simulink model "SAR_Heavy_Mapper_SITL_3D_v1"  (R2025b)
settings: Solver=ode4  StartTime=0.0  StopTime=inf  FixedStep=1/60  RelTol=1e-3
libraries: dspnetwork x4, sim3dlib x1, uavsim3dlib x1
settings Model: Creator=User  LastModifiedBy=User

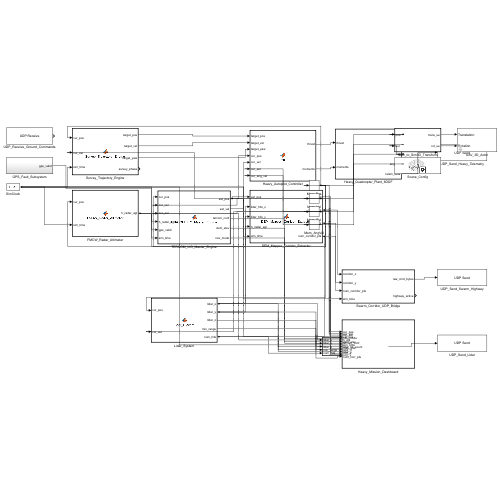
[thumbnail: Simulink's stored preview of the top-level diagram]
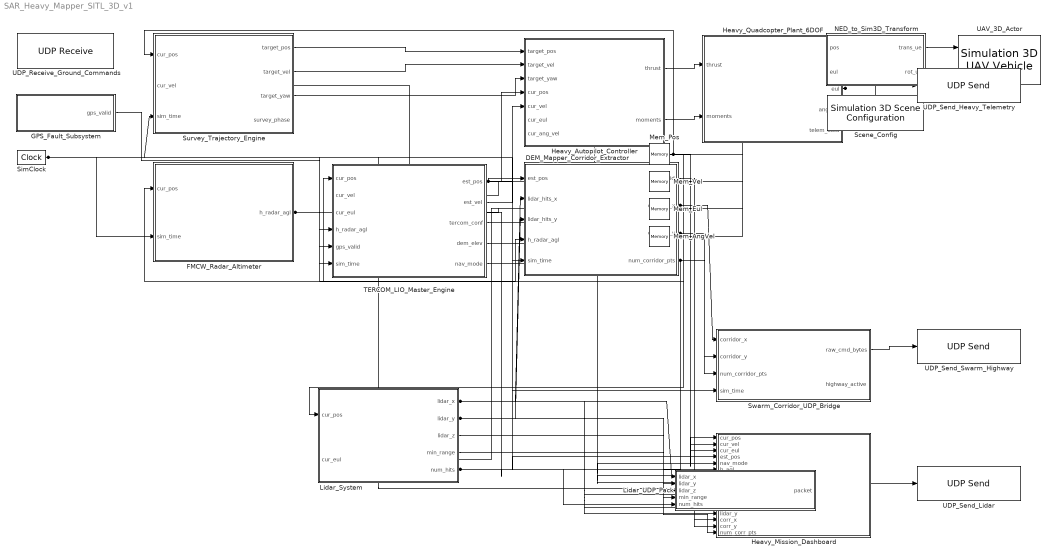
== system SAR_Heavy_Mapper_SITL_3D_v1 ==
  DEM_Mapper_Corridor_Extractor : MATLAB Function  TreatAsAtomicUnit=on
  FMCW_Radar_Altimeter : MATLAB Function  TreatAsAtomicUnit=on
  GPS_Fault_Subsystem : Subsystem
  Heavy_Autopilot_Controller : MATLAB Function  TreatAsAtomicUnit=on
  Heavy_Mission_Dashboard : MATLAB Function  TreatAsAtomicUnit=on
  Heavy_Quadcopter_Plant_6DOF : MATLAB Function  TreatAsAtomicUnit=on
  Lidar_System : MATLAB Function  TreatAsAtomicUnit=on
  Lidar_UDP_Pack : MATLAB Function  TreatAsAtomicUnit=on
  Mem_AngVel : Memory  InitialCondition=[0; 0; 0]
  Mem_Eul : Memory  InitialCondition=[0; 0; 0]
  Mem_Pos : Memory  InitialCondition=[0; 0; -70]
  Mem_Vel : Memory  InitialCondition=[0; 0; 0]
  NED_to_Sim3D_Transform : MATLAB Function  TreatAsAtomicUnit=on
  Scene_Config : sim3dlib/Simulation 3D Scene Configuration  Priority=0  ProjectFormat=Default Scenes  SceneDesc=US city block  ProjectName=D:\MLAB\toolbox\shared\sim3d_projects\automotive_project_windows\UE\WindowsNoEditor\VehicleSimulation.exe  ScenePath=/Game/Maps/USCityBlock  EnableOpenDRIVE=off  vehTagList={'Custom';'Scene Origin'}  vehTag=Scene Origin  AttachedCameraRelativeTranslation=[0 0 0]  FreeCameraDefaultInitialTranslation=[-6, 0, 2]  AttachedCameraRelativeRotation=[0 0 0]  FreeCameraDefaultInitialRotation=[0, -15, 0]  ViewpointName=Custom  FreeCameraInitialTranslation=[0, 0, 0]  ViewpointTranslation=[0, 0, 0]  FreeCameraInitialRotation=[0, 0, 0]  ViewpointRotation=[0, 0, 0]  OpVisEn=off  Ts=1/60  EnableWindow=on  EnableRemoteAccess=off  EnableWeather=off  SunAzimuth=90  SunAltitude=40.0  EnableGeospatialSun=off  Latitude=0  Longitude=0  Date=2023-01-01  Time=10:30:00  GeoTimeZone=-5.0  SunDaylightSaving=off  wind=1  clouds=10  EnableVolumetricClouds=off  CloudCoverage=0  CloudAltitude=6  fog=0  rain=0  RaindropsEffect=off  SnowDensity=0  EnableGeospatial=off  TilesetSource=Earth terrain  UseTrueOrigin=off  OriginHeight=200  OriginLatitude=40.744652  OriginLongitude=-73.988864  MapStyle=Aerial  AdditionalAssetIDs=[]  UseAdvancedSunSky=off  SolarTime=11  TimeZone=-5  Day=21  Month=9  Year=2022  UseDaylightSavingTime=on  DSTStartDay=10  DSTStartMonth=3  DSTEndDay=3  DSTEndMonth=11  DSTSwitchHour=2  sensorTag=MainCamera1  sensorId=1  sensorName=MainCamera1  mountLoc=Origin  offsetFlag=off  tmountOffset=[0, 0, 0]  rmountOffset=[0, 0, 0]  HorizontalResolution=1280  VerticalResolution=720  HorizontalFOV=60  mountPoint=[0 0 0]  mountOrientation=[0 0 0]  aMode=4  ID=1  GeoTrigger=Inactive  ViewNameList={'Custom'}  ViewTranslationList={'[0 0 0]'}  ViewRotationList={'[0 0 0]'}
      settings: LibrarySourceBlock=uavsim3dlib/Simulation 3D Scene Configuration
  SimClock : DigitalClock  SampleTime=1/60
  Survey_Trajectory_Engine : MATLAB Function  TreatAsAtomicUnit=on
  Swarm_Corridor_UDP_Bridge : MATLAB Function  TreatAsAtomicUnit=on
  TERCOM_LIO_Master_Engine : MATLAB Function  TreatAsAtomicUnit=on
  UAV_3D_Actor : uavsim3dlib/Simulation 3D UAV Vehicle  Priority=-1  Mesh=Quadrotor  MeshPath=/MathWorksUAVContent/UAVs/HexaRotorUAV/HexaRotor.HexaRotor  Color=Black  ActorName=SimulinkVehicle1  UseGlobalFrame=off  InitialTranslation=[0 0 0]  InitialRotation=[0 0 0]  InitialTranslationGlobal=[0 0 0]  InitialGeoOrigin=[0 0 0]  InitialRotationGlobal=[0 0 0]  SampleTime=-1  ActorType=SimulinkVehicle  ID=1  aMode=4  ActorTag=SimulinkVehicle1
  UDP_Receive_Ground_Commands : dspnetwork/UDP Receive  localURL='0.0.0.0'  localPort=6001  remoteURL='0.0.0.0'  remotePort=-1  recvBufferSize=8192  dims=255  signalDatatype=uint8  isComplex=off  isVarSize=on  showBlockingTime=off  blockingTime=0  sampletime=1  blockPlatform=[]
  UDP_Send_Heavy_Telemetry : dspnetwork/UDP Send  remoteURL='127.0.0.1'  remotePort=6002  localURL='0.0.0.0'  localPortSource=Automatically determine  localPort=2048  sendBufferSize=8192  sampletime=-1  blockPlatform=[]  separateLengthPort=0
  UDP_Send_Lidar : dspnetwork/UDP Send  remoteURL='127.0.0.1'  remotePort=5003  localURL='0.0.0.0'  localPortSource=Automatically determine  localPort=2048  sendBufferSize=8192  sampletime=-1  blockPlatform=[]  separateLengthPort=0
  UDP_Send_Swarm_Highway : dspnetwork/UDP Send  remoteURL='127.0.0.1'  remotePort=5001  localURL='0.0.0.0'  localPortSource=Automatically determine  localPort=2048  sendBufferSize=8192  sampletime=-1  blockPlatform=[]  separateLengthPort=0
  wires:
  Mem_Pos/1 -> Survey_Trajectory_Engine/1(cur_pos), FMCW_Radar_Altimeter/1(cur_pos), TERCOM_LIO_Master_Engine/1(cur_pos), Lidar_System/1(cur_pos), Heavy_Mission_Dashboard/1(cur_pos)
  Mem_Vel/1 -> Survey_Trajectory_Engine/2(cur_vel), TERCOM_LIO_Master_Engine/2(cur_vel), Heavy_Mission_Dashboard/2(cur_vel)
  SimClock/1 -> Survey_Trajectory_Engine/3(sim_time), FMCW_Radar_Altimeter/2(sim_time), TERCOM_LIO_Master_Engine/6(sim_time), DEM_Mapper_Corridor_Extractor/5(sim_time), Swarm_Corridor_UDP_Bridge/4(sim_time), Heavy_Mission_Dashboard/9(sim_time)
  Mem_Eul/1 -> TERCOM_LIO_Master_Engine/3(cur_eul), Lidar_System/2(cur_eul), Heavy_Autopilot_Controller/6(cur_eul), Heavy_Mission_Dashboard/3(cur_eul)
  FMCW_Radar_Altimeter/1(h_radar_agl) -> TERCOM_LIO_Master_Engine/4(h_radar_agl), DEM_Mapper_Corridor_Extractor/4(h_radar_agl), Heavy_Mission_Dashboard/6(h_agl)
  GPS_Fault_Subsystem/1(gps_valid) -> TERCOM_LIO_Master_Engine/5(gps_valid)
  Lidar_System/1(lidar_x) -> Lidar_UDP_Pack/1(lidar_x), DEM_Mapper_Corridor_Extractor/2(lidar_hits_x), Heavy_Mission_Dashboard/12(lidar_x)
  Lidar_System/2(lidar_y) -> Lidar_UDP_Pack/2(lidar_y), DEM_Mapper_Corridor_Extractor/3(lidar_hits_y), Heavy_Mission_Dashboard/13(lidar_y)
  Lidar_System/3(lidar_z) -> Lidar_UDP_Pack/3(lidar_z)
  Lidar_System/4(min_range) -> Lidar_UDP_Pack/4(min_range)
  Lidar_System/5(num_hits) -> Lidar_UDP_Pack/5(num_hits), Heavy_Mission_Dashboard/10(lidar_hit_count)
  Lidar_UDP_Pack/1(packet) -> UDP_Send_Lidar/1
  TERCOM_LIO_Master_Engine/1(est_pos) -> DEM_Mapper_Corridor_Extractor/1(est_pos), Heavy_Autopilot_Controller/4(cur_pos), Heavy_Mission_Dashboard/4(est_pos)
  DEM_Mapper_Corridor_Extractor/2(corridor_x) -> Swarm_Corridor_UDP_Bridge/1(corridor_x), Heavy_Mission_Dashboard/14(corr_x)
  DEM_Mapper_Corridor_Extractor/3(corridor_y) -> Swarm_Corridor_UDP_Bridge/2(corridor_y), Heavy_Mission_Dashboard/15(corr_y)
  DEM_Mapper_Corridor_Extractor/4(num_corridor_pts) -> Swarm_Corridor_UDP_Bridge/3(num_corridor_pts), Heavy_Mission_Dashboard/16(num_corr_pts)
  Swarm_Corridor_UDP_Bridge/1(raw_cmd_bytes) -> UDP_Send_Swarm_Highway/1
  Survey_Trajectory_Engine/1(target_pos) -> Heavy_Autopilot_Controller/1(target_pos)
  Survey_Trajectory_Engine/2(target_vel) -> Heavy_Autopilot_Controller/2(target_vel)
  Survey_Trajectory_Engine/3(target_yaw) -> Heavy_Autopilot_Controller/3(target_yaw)
  TERCOM_LIO_Master_Engine/2(est_vel) -> Heavy_Autopilot_Controller/5(cur_vel)
  Mem_AngVel/1 -> Heavy_Autopilot_Controller/7(cur_ang_vel)
  Heavy_Autopilot_Controller/1(thrust) -> Heavy_Quadcopter_Plant_6DOF/1(thrust)
  Heavy_Autopilot_Controller/2(moments) -> Heavy_Quadcopter_Plant_6DOF/2(moments)
  Heavy_Quadcopter_Plant_6DOF/1(pos) -> Mem_Pos/1, NED_to_Sim3D_Transform/1(pos)
  Heavy_Quadcopter_Plant_6DOF/2(vel) -> Mem_Vel/1
  Heavy_Quadcopter_Plant_6DOF/3(eul) -> Mem_Eul/1, NED_to_Sim3D_Transform/2(eul)
  Heavy_Quadcopter_Plant_6DOF/4(ang_vel) -> Mem_AngVel/1
  Heavy_Quadcopter_Plant_6DOF/5(telem_data) -> UDP_Send_Heavy_Telemetry/1
  NED_to_Sim3D_Transform/1(trans_ue) -> UAV_3D_Actor/1
  NED_to_Sim3D_Transform/2(rot_ue) -> UAV_3D_Actor/2
  TERCOM_LIO_Master_Engine/5(nav_mode) -> Heavy_Mission_Dashboard/5(nav_mode)
  TERCOM_LIO_Master_Engine/4(dem_elev) -> Heavy_Mission_Dashboard/7(dem_elev)
  TERCOM_LIO_Master_Engine/3(tercom_conf) -> Heavy_Mission_Dashboard/8(tercom_conf)
  DEM_Mapper_Corridor_Extractor/1(map_grid) -> Heavy_Mission_Dashboard/11(map_grid)

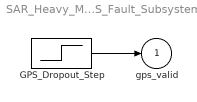
== system SAR_Heavy_Mapper_SITL_3D_v1/GPS_Fault_Subsystem ==
  GPS_Dropout_Step : Step  Time=60  Before=1  After=0  SampleTime=1/60
  gps_valid : Outport
  wires:
  ? -> ?
  GPS_Dropout_Step/1 -> gps_valid/1

== matlab function SAR_Heavy_Mapper_SITL_3D_v1/Heavy_Autopilot_Controller ==
  data: target_pos input; thrust output size=1; target_vel input; target_yaw input; cur_pos input; cur_vel input; cur_eul input; cur_ang_vel input; moments output size=3
function [thrust, moments] = Heavy_Autopilot_Controller(target_pos, target_vel, target_yaw, cur_pos, cur_vel, cur_eul, cur_ang_vel)
thrust = 0.0; moments = [0.0; 0.0; 0.0];
persistent int_vel_err int_z_err pitch_cmd_filt roll_cmd_filt
if isempty(int_vel_err)
    int_vel_err = [0; 0]; int_z_err = 0.0;
    pitch_cmd_filt = 0.0; roll_cmd_filt = 0.0;
end
dt = 1/60; m = 9.5; g = 9.81;

kp_p = 1.4; kp_v = 2.8; ki_v = 0.08;
e_pos = target_pos(1:2) - cur_pos(1:2);
e_vel = target_vel(1:2) - cur_vel(1:2);
int_vel_err = max(min(int_vel_err + (e_vel * dt), 1.5), -1.5);
acc_world = kp_p * e_pos + kp_v * e_vel + ki_v * int_vel_err;

yaw = cur_eul(3);
acc_bx =  acc_world(1) * cos(yaw) + acc_world(2) * sin(yaw);
acc_by = -acc_world(1) * sin(yaw) + acc_world(2) * cos(yaw);

MAX_TILT = 18.0 * pi / 180.0;
pitch_cmd = max(min(-acc_bx / g, MAX_TILT), -MAX_TILT);
roll_cmd  = max(min( acc_by / g, MAX_TILT), -MAX_TILT);

alpha = 0.12;
pitch_cmd_filt = (1.0 - alpha) * pitch_cmd_filt + alpha * pitch_cmd;
roll_cmd_filt  = (1.0 - alpha) * roll_cmd_filt  + alpha * roll_cmd;

kp_z = 8.5; kd_z = 4.2; ki_z = 0.4;
e_z = target_pos(3) - cur_pos(3);
e_vz = target_vel(3) - cur_vel(3);
int_z_err = max(min(int_z_err + e_z * dt, 2.0), -2.0);
az_cmd = kp_z * e_z + kd_z * e_vz + ki_z * int_z_err;

cos_tilt = max(0.75, cos(cur_eul(1)) * cos(cur_eul(2)));
thrust = m * (g - az_cmd) / cos_tilt;
thrust = max(0.3 * m * g, min(thrust, 2.5 * m * g));

kp_att = [12.0; 12.0; 6.0];
kd_att = [1.2; 1.2; 0.8];
yaw_tgt_rad = target_yaw * pi / 180.0;
yaw_err = atan2(sin(yaw_tgt_rad - cur_eul(3)), cos(yaw_tgt_rad - cur_eul(3)));
att_err = [roll_cmd_filt - cur_eul(1); pitch_cmd_filt - cur_eul(2); yaw_err];
moments = kp_att .* att_err - kd_att .* cur_ang_vel;

== matlab function SAR_Heavy_Mapper_SITL_3D_v1/Heavy_Quadcopter_Plant_6DOF ==
  data: thrust input; pos output size=3; moments input; vel output size=3; eul output size=3; ang_vel output size=3; telem_data output size=16
function [pos, vel, eul, ang_vel, telem_data] = Heavy_Quadcopter_Plant_6DOF(thrust, moments)
pos = zeros(3, 1); vel = zeros(3, 1); eul = zeros(3, 1); ang_vel = zeros(3, 1); telem_data = zeros(16, 1);
persistent p v e w
if isempty(p)
    p = [0; 0; -70]; % Initialize at 70m survey vantage
    v = [0; 0; 0]; e = [0; 0; 0]; w = [0; 0; 0];
end
dt = 1/60; m = 9.5; g = 9.81;
I = diag([0.22, 0.22, 0.42]);

phi = e(1); theta = e(2); psi = e(3);
R = [cos(theta)*cos(psi), sin(phi)*sin(theta)*cos(psi)-cos(phi)*sin(psi), cos(phi)*sin(theta)*cos(psi)+sin(phi)*sin(psi);
     cos(theta)*sin(psi), sin(phi)*sin(theta)*sin(psi)+cos(phi)*cos(psi), cos(phi)*sin(theta)*sin(psi)-sin(phi)*cos(psi);
    -sin(theta),          sin(phi)*cos(theta),                            cos(phi)*cos(theta)];

f_body = [0; 0; -thrust];
drag = -0.15 * norm(v(1:2)) * [v(1); v(2); 0];
acc = (R * f_body + [0; 0; m*g] + drag) / m;
v = v + acc * dt; p = p + v * dt;

ang_acc = I \ (moments - cross(w, I * w));
w = w + ang_acc * dt;
T = [1, sin(phi)*tan(theta), cos(phi)*tan(theta); 0, cos(phi), -sin(phi); 0, sin(phi)/cos(theta), cos(phi)/cos(theta)];
e = e + (T * w) * dt;
e(3) = atan2(sin(e(3)), cos(e(3)));

pos = p; vel = v; eul = e; ang_vel = w;
telem_data(1:3) = p; telem_data(4:6) = v; telem_data(7:9) = e;
telem_data(10)  = thrust;

== matlab function SAR_Heavy_Mapper_SITL_3D_v1/NED_to_Sim3D_Transform ==
  data: pos input; trans_ue output size=3; eul input; rot_ue output size=3
function [trans_ue, rot_ue] = NED_to_Sim3D_Transform(pos, eul)
trans_ue = zeros(3, 1);
rot_ue   = zeros(3, 1);
trans_ue(1) = pos(1);
trans_ue(2) = -pos(2);
trans_ue(3) = -pos(3);
rot_ue(1) = -eul(3);
rot_ue(2) = -eul(2);
rot_ue(3) =  eul(1);

== matlab function SAR_Heavy_Mapper_SITL_3D_v1/Heavy_Mission_Dashboard ==
  data: cur_pos input; cur_vel input; cur_eul input; est_pos input; nav_mode input; h_agl input; dem_elev input; tercom_conf input; sim_time input; lidar_hit_count input; map_grid input; lidar_x input; lidar_y input; corr_x input; corr_y input; num_corr_pts input
function Heavy_Mission_Dashboard(cur_pos, cur_vel, cur_eul, est_pos, nav_mode, h_agl, dem_elev, tercom_conf, sim_time, lidar_hit_count, map_grid, lidar_x, lidar_y, corr_x, corr_y, num_corr_pts)
coder.extrinsic('heavyMapperDashboardLivePlot');
heavyMapperDashboardLivePlot(cur_pos, cur_vel, cur_eul, est_pos, nav_mode, h_agl, dem_elev, tercom_conf, sim_time, lidar_hit_count, map_grid, lidar_x, lidar_y, corr_x, corr_y, num_corr_pts);

== matlab function SAR_Heavy_Mapper_SITL_3D_v1/Lidar_System ==
  data: cur_pos input; lidar_x output size=108; cur_eul input; lidar_y output size=108; lidar_z output size=108; min_range output size=1; num_hits output size=1
function [lidar_x, lidar_y, lidar_z, min_range, num_hits] = Lidar_System(cur_pos, cur_eul)
N_AZ = 36; ELEVS = [30, 55, 80] * pi / 180; N_EL = numel(ELEVS); N = N_AZ * N_EL;
MAX_RANGE = 150.0; % High-altitude 150m survey envelope
lidar_x = zeros(N, 1); lidar_y = zeros(N, 1); lidar_z = zeros(N, 1);
min_range = MAX_RANGE; num_hits = 0.0;
persistent buildings
if isempty(buildings)
    buildings = [
        -12.5,  46.0,   8.0,  80.0, -35.0, 0.0;   % Northwest Block 1
         54.0, 111.0,   8.0,  80.0, -35.0, 0.0;   % Northwest Block 2 (Red brick building)
        -12.5,  46.0, -80.0,  -8.0, -35.0, 0.0;   % Southwest Block 1
         54.0, 111.0, -80.0,  -8.0, -35.0, 0.0;   % Southwest Block 2
        195.0, 255.0,   8.0,  80.0, -35.0, 0.0;   % Far East Block
        129.0, 200.0, -80.0,  -8.0, -35.0, 0.0;   % Southeast Block
        -80.0, -29.0,   8.0,  80.0, -35.0, 0.0;   % West-North Block
        -80.0, -29.0, -80.0,  -8.0, -35.0, 0.0    % West-South Block
    ];
end

az_body = (-pi + (0:N_AZ-1) * (2*pi/N_AZ))';
az_rep = repmat(az_body, N_EL, 1); el_rep = repelem(ELEVS(:), N_AZ);
dx_b = cos(az_rep) .* cos(el_rep); dy_b = sin(az_rep) .* cos(el_rep); dz_b = sin(el_rep);

yaw = cur_eul(3); c = cos(yaw); s = sin(yaw);
dx_w = c * dx_b - s * dy_b; dy_w = s * dx_b + c * dy_b; dz_w = dz_b;

ox = cur_pos(1); oy = cur_pos(2); oz = cur_pos(3);
best_t = MAX_RANGE * ones(N, 1); hit_flags = false(N, 1);

% Ground Plane Intersection (z = 0)
for r = 1:N
    if dz_w(r) > 0.05
        t_g = -oz / dz_w(r);
        if t_g > 0.0 && t_g < best_t(r)
            best_t(r) = t_g; hit_flags(r) = true;
        end
    end
end

% 3D Building Facade & Roof Intersections
for r = 1:N
    rx = dx_w(r); ry = dy_w(r); rz = dz_w(r);
    for b = 1:size(buildings, 1)
        bx1 = buildings(b, 1); bx2 = buildings(b, 2);
        by1 = buildings(b, 3); by2 = buildings(b, 4);
        bz1 = buildings(b, 5); bz2 = buildings(b, 6);
        if abs(rx) > 1e-5; tx1 = (bx1 - ox) / rx; tx2 = (bx2 - ox) / rx;
        else; tx1 = -1e6; tx2 = 1e6; end
        if abs(ry) > 1e-5; ty1 = (by1 - oy) / ry; ty2 = (by2 - oy) / ry;
        else; ty1 = -1e6; ty2 = 1e6; end
        if abs(rz) > 1e-5; tz1 = (bz1 - oz) / rz; tz2 = (bz2 - oz) / rz;
        else; tz1 = -1e6; tz2 = 1e6; end
        tmin_x = min(tx1, tx2); tmax_x = max(tx1, tx2);
        tmin_y = min(ty1, ty2); tmax_y = max(ty1, ty2);
        tmin_z = min(tz1, tz2); tmax_z = max(tz1, tz2);
        t_enter = max(max(tmin_x, tmin_y), tmin_z);
        t_exit  = min(min(tmax_x, tmax_y), tmax_z);
        if t_exit >= max(0.0, t_enter) && t_enter < best_t(r)
            best_t(r) = t_enter; hit_flags(r) = true;
        end
    end
end

lidar_x = best_t .* dx_b;
lidar_y = best_t .* dy_b;
lidar_z = best_t .* dz_b;
num_hits = double(sum(hit_flags));
if any(hit_flags); min_range = min(best_t(hit_flags)); else; min_range = MAX_RANGE; end

== matlab function SAR_Heavy_Mapper_SITL_3D_v1/Survey_Trajectory_Engine ==
  data: cur_pos input; target_pos output size=3; cur_vel input; sim_time input; target_vel output size=3; target_yaw output size=1; survey_phase output size=1
function [target_pos, target_vel, target_yaw, survey_phase] = Survey_Trajectory_Engine(cur_pos, cur_vel, sim_time)
target_pos = zeros(3, 1); target_vel = zeros(3, 1); target_yaw = 0.0; survey_phase = 1.0;
persistent wps wp_idx is_init
CRUISE_ALT = -70.0; % High-altitude vantage (70 m AGL)
if isempty(is_init)
    is_init = true; wp_idx = 1.0;
    wps = [
        0.0,    0.0,   CRUISE_ALT;
        220.0,  0.0,   CRUISE_ALT;
        220.0,  30.0,  CRUISE_ALT;
        -30.0,  30.0,  CRUISE_ALT;
        -30.0,  60.0,  CRUISE_ALT;
        220.0,  60.0,  CRUISE_ALT;
        220.0, -30.0,  CRUISE_ALT;
        -30.0, -30.0,  CRUISE_ALT
    ];
end
c_idx = int32(wp_idx);
tgt = wps(c_idx, :)';
d_err = norm(tgt(1:2) - cur_pos(1:2));
if d_err < 6.0
    wp_idx = double(mod(c_idx, int32(size(wps, 1))) + 1);
    tgt = wps(int32(wp_idx), :)';
end
V_SURVEY = 8.5;
dir_xy = tgt(1:2) - cur_pos(1:2);
if norm(dir_xy) > 0.1; dir_xy = dir_xy / norm(dir_xy); end
target_pos = tgt;
target_vel = [dir_xy(1) * V_SURVEY; dir_xy(2) * V_SURVEY; 0.0];
target_yaw = atan2(dir_xy(2), dir_xy(1)) * 180.0 / pi;

== matlab function SAR_Heavy_Mapper_SITL_3D_v1/Lidar_UDP_Pack ==
  data: lidar_x input; packet output size=327; lidar_y input; lidar_z input; min_range input; num_hits input
function packet = Lidar_UDP_Pack(lidar_x, lidar_y, lidar_z, min_range, num_hits)
packet = [double(numel(lidar_x)); lidar_x(:); lidar_y(:); lidar_z(:); double(min_range); double(num_hits)];

== matlab function SAR_Heavy_Mapper_SITL_3D_v1/FMCW_Radar_Altimeter ==
  data: cur_pos input; h_radar_agl output size=1; sim_time input
function h_radar_agl = FMCW_Radar_Altimeter(cur_pos, sim_time)
x = cur_pos(1); y = cur_pos(2);
z_ground = 7.5 * sin(0.025 * x) * cos(0.025 * y) + 3.2 * sin(0.06 * x);
true_agl = max(0.0, -cur_pos(3) - z_ground);
h_radar_agl = true_agl + 0.05 * sin(sim_time * 15.0);

== matlab function SAR_Heavy_Mapper_SITL_3D_v1/TERCOM_LIO_Master_Engine ==
  data: cur_pos input; est_pos output size=3; cur_vel input; cur_eul input; h_radar_agl input; gps_valid input; sim_time input; est_vel output size=3; tercom_conf output size=1; dem_elev output size=1; nav_mode output size=1
function [est_pos, est_vel, tercom_conf, dem_elev, nav_mode] = TERCOM_LIO_Master_Engine(cur_pos, cur_vel, cur_eul, h_radar_agl, gps_valid, sim_time)
est_pos = [0.0; 0.0; 0.0]; est_vel = [0.0; 0.0; 0.0]; tercom_conf = 0.95; dem_elev = 0.0; nav_mode = 0.0;
persistent p_est v_est P_cov last_time buffer_prof
if isempty(P_cov)
    p_est = cur_pos; v_est = cur_vel;
    P_cov = blkdiag(0.2*eye(3), 0.05*eye(3));
    last_time = sim_time;
    buffer_prof = zeros(15, 1);
end
dt = sim_time - last_time;
if dt <= 0 || dt > 0.1; dt = 1/60; end
last_time = sim_time;

meas_ground_elev = -cur_pos(3) - h_radar_agl;
dem_elev = meas_ground_elev;
buffer_prof = [buffer_prof(2:end); meas_ground_elev];

terrain_variance = var(buffer_prof);
is_flat = (terrain_variance < 0.12);

if gps_valid >= 0.5
    nav_mode = 0.0; % GPS Primary
    p_est = cur_pos; v_est = cur_vel;
    tercom_conf = 0.98;
elseif ~is_flat
    nav_mode = 1.0; % BATCH TERCOM MATCHING ACTIVE
    expected_elev = 7.5 * sin(0.025 * p_est(1)) * cos(0.025 * p_est(2)) + 3.2 * sin(0.06 * p_est(1));
    elev_resid = meas_ground_elev - expected_elev;
    p_est(1) = p_est(1) + 0.15 * elev_resid;
    p_est(2) = p_est(2) + 0.15 * elev_resid;
    p_est(3) = cur_pos(3);
    v_est = cur_vel;
    tercom_conf = max(0.65, min(0.96, 1.0 - abs(elev_resid) / 8.0));
else
    nav_mode = 2.0; % FLAT TERRAIN CONTINGENCY: FALLBACK TO TIGHT LIO
    p_est = p_est + v_est * dt;
    v_est = cur_vel;
    tercom_conf = 0.55;
end
est_pos = p_est; est_vel = v_est;

== matlab function SAR_Heavy_Mapper_SITL_3D_v1/DEM_Mapper_Corridor_Extractor ==
  data: est_pos input; map_grid output size=625; lidar_hits_x input; lidar_hits_y input; h_radar_agl input; sim_time input; corridor_x output size=16; corridor_y output size=16; num_corridor_pts output size=1
function [map_grid, corridor_x, corridor_y, num_corridor_pts] = DEM_Mapper_Corridor_Extractor(est_pos, lidar_hits_x, lidar_hits_y, h_radar_agl, sim_time)
map_grid = zeros(625, 1);
corridor_x = zeros(16, 1); corridor_y = zeros(16, 1); num_corridor_pts = 4.0;
persistent grid_accum
if isempty(grid_accum)
    grid_accum = zeros(25, 25);
end

gx = linspace(-50, 250, 25); gy = linspace(-100, 100, 25);
for i = 1:numel(gx)
    for j = 1:numel(gy)
        grid_accum(i, j) = 7.5 * sin(0.025 * gx(i)) * cos(0.025 * gy(j)) + 3.2 * sin(0.06 * gx(i));
    end
end
map_grid = grid_accum(:);

corridor_x(1) = 0.0;   corridor_y(1) = 0.0;
corridor_x(2) = 60.0;  corridor_y(2) = 15.0;
corridor_x(3) = 135.0; corridor_y(3) = 15.0;
corridor_x(4) = 180.0; corridor_y(4) = 45.0;
num_corridor_pts = 4.0;

== matlab function SAR_Heavy_Mapper_SITL_3D_v1/Swarm_Corridor_UDP_Bridge ==
  data: corridor_x input; raw_cmd_bytes output size=18; corridor_y input; num_corridor_pts input; sim_time input; highway_active output size=1
function [raw_cmd_bytes, highway_active] = Swarm_Corridor_UDP_Bridge(corridor_x, corridor_y, num_corridor_pts, sim_time)
raw_cmd_bytes = zeros(18, 1, 'uint8');
highway_active = 1.0;

raw_cmd_bytes(1) = uint8(170);
raw_cmd_bytes(2) = uint8(3);

p1 = single(corridor_x(3));
p2 = single(corridor_y(3));
p3 = single(-15.0);
p4 = single(0.0);

b1 = typecast(p1, 'uint8'); b2 = typecast(p2, 'uint8');
b3 = typecast(p3, 'uint8'); b4 = typecast(p4, 'uint8');
for i = 1:4
    raw_cmd_bytes(2 + i)  = b1(i);
    raw_cmd_bytes(6 + i)  = b2(i);
    raw_cmd_bytes(10 + i) = b3(i);
    raw_cmd_bytes(14 + i) = b4(i);
end
